simulink model "untitled"  (R2022b)
settings: Solver=VariableStepAuto  StartTime=0.0  StopTime=100  RelTol=1e-3
settings Model: Creator=serez  LastModifiedBy=serez

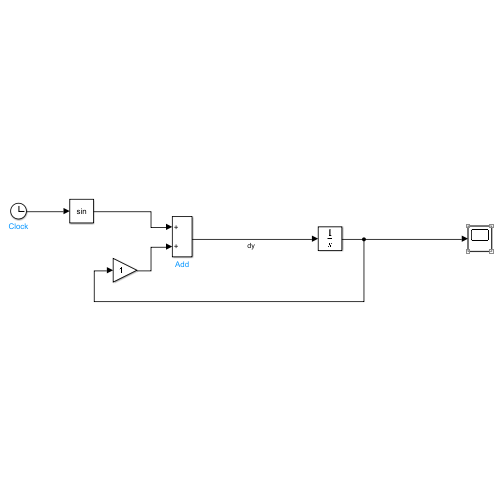
[thumbnail: Simulink's stored preview of the top-level diagram]
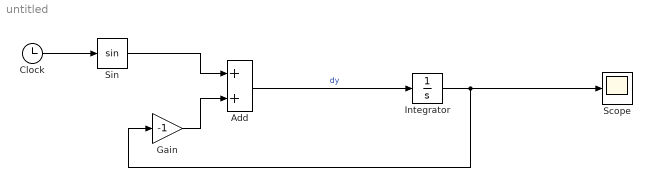
== system untitled ==
  Add : Sum
  Clock : Clock
  Gain : Gain  Gain=-1
  Integrator : Integrator
  Scope : Scope
  Sin : Trigonometry
  wires:
  Clock/1 -> Sin/1
  Sin/1 -> Add/1
  Gain/1 -> Add/2
  Add/1 -> Integrator/1  "dy"
  Integrator/1 -> Gain/1, Scope/1
